simulink model "Capitol7Pb1"  (R2013a)
settings: Solver=ode45  StartTime=0.0  StopTime=50.0  RelTol=1e-3
undefined symbols (not defined in the file): des, gcbh
settings Model: Creator=user  LastModifiedBy=user

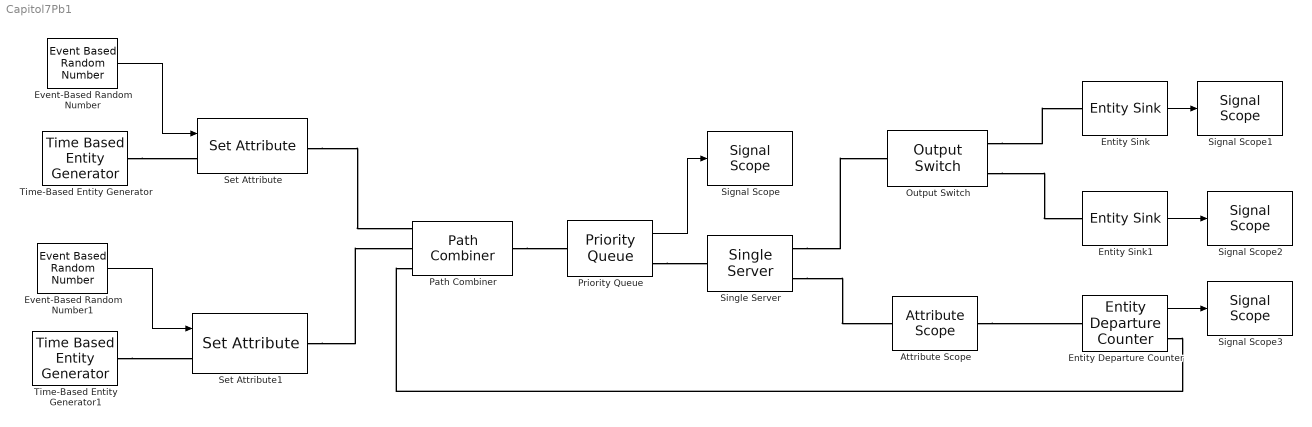
== system Capitol7Pb1 ==
  Attribute Scope : AttributeScope  LoadFcn=des.scope.CallbackSupport('seLoadFcn',gcbh)  StartFcn=des.scope.CallbackSupport('seStartFcn',gcbh)  StopFcn=des.scope.CallbackSupport('seStopFcn',gcbh)  AttributeNameY=ServiceTime
      settings: CopyFcn=des.scope.CallbackSupport('seCopyFcn',gcbh)  DeleteFcn=des.scope.CallbackSupport('seDeleteFcn',gcbh)  PreSaveFcn=des.scope.CallbackSupport('sePreSaveFcn',gcbh)  NameChangeFcn=des.scope.CallbackSupport('seNameChangeFcn',gcbh)  OpenFcn=des.scope.CallbackSupport('seOpenFcn',gcbh)
  Entity Departure Counter : EntityDepartureCounter  NumberDepartedToSignal=on
  Entity Sink : EntitySink  StatNumberArrived=on
  Entity Sink1 : EntitySink  StatNumberArrived=on
  Event-Based Random Number : EventBasedRandomNumber
  Event-Based Random Number1 : EventBasedRandomNumber  meanExp=2.5
  Output Switch : OutputSwitch  NumberOutputPorts=2
  Path Combiner : PathCombiner
  Priority Queue : PriorityQueue  SortingAttributeName=Preedmted  StatAverageQueueLength=on
      settings: OutputPortMap=o3
  Set Attribute : SetAttribute  AttributeName=Type|ServiceTime|Priority|Preedmted  AttributeFrom=Dialog|Signal port|Dialog|Dialog  AttributeValue=1|1|1|0  AttributeTreatAsVector=1|1|1|1  EvaluatedAttributeValue={ 1;[];1;0}
      settings: InputPortMap=u1
  Set Attribute1 : SetAttribute  AttributeName=Type|ServiceTime|Priority|Preedmted  AttributeFrom=Dialog|Signal port|Dialog|Dialog  AttributeValue=2|1|2|0  AttributeTreatAsVector=1|1|1|1  EvaluatedAttributeValue={ 2;[];2;0}
      settings: InputPortMap=u1
  Signal Scope{,1..3} (4 alike) : SignalScope  LoadFcn=des.scope.CallbackSupport('seLoadFcn',gcbh)  StartFcn=des.scope.CallbackSupport('seStartFcn',gcbh)  StopFcn=des.scope.CallbackSupport('seStopFcn',gcbh)
      settings: CopyFcn=des.scope.CallbackSupport('seCopyFcn',gcbh)  DeleteFcn=des.scope.CallbackSupport('seDeleteFcn',gcbh)  PreSaveFcn=des.scope.CallbackSupport('sePreSaveFcn',gcbh)  NameChangeFcn=des.scope.CallbackSupport('seNameChangeFcn',gcbh)  OpenFcn=des.scope.CallbackSupport('seOpenFcn',gcbh)
  Single Server : SingleServer  ServiceTimeFrom=Attribute  PermitPreemption=on  SortingAttributeName=Priority  WriteToAttribute=on  ResidualAttributeName=ServiceTime
  Time-Based Entity Generator : TimeBasedEntityGenerator  Period=2
  Time-Based Entity Generator1 : TimeBasedEntityGenerator  Period=5
  wires:
  Priority Queue/1 -> Signal Scope/1
  Entity Sink/1 -> Signal Scope1/1
  Entity Sink1/1 -> Signal Scope2/1
  Event-Based Random Number/1 -> Set Attribute/1
  Event-Based Random Number1/1 -> Set Attribute1/1
  Entity Departure Counter/1 -> Signal Scope3/1
  connections:
  Time-Based Entity Generator/RConn1 -- Set Attribute/LConn1
  Time-Based Entity Generator1/RConn1 -- Set Attribute1/LConn1
  Set Attribute/RConn1 -- Path Combiner/LConn1
  Set Attribute1/RConn1 -- Path Combiner/LConn2
  Path Combiner/RConn1 -- Priority Queue/LConn1
  Priority Queue/RConn1 -- Single Server/LConn1
  Single Server/RConn1 -- Output Switch/LConn1
  Output Switch/RConn1 -- Entity Sink/LConn1
  Output Switch/RConn2 -- Entity Sink1/LConn1
  Single Server/RConn2 -- Attribute Scope/LConn1
  Attribute Scope/RConn1 -- Entity Departure Counter/LConn1
  Entity Departure Counter/RConn1 -- Path Combiner/LConn3
